simulink model "virtualWallSim"  (Simulink 8.1)
settings: Solver=ode45  StartTime=0.0  StopTime=5  MaxStep=0.01  RelTol=1e-3
libraries: simulink x1
settings Model: Creator=jasonyt  LastModifiedBy=jasonyt
settings DataIOCC: LimitDataPoints=off  SignalLoggingSaveFormat=Dataset
settings OptimizationCC: ExpressionDepthLimit=128
settings DebuggingCC: FcnCallInpInsideContextMsg=EnableAllAsError
settings GRTTargetCC: CombineOutputUpdateFcns=on  GRTInterface=off

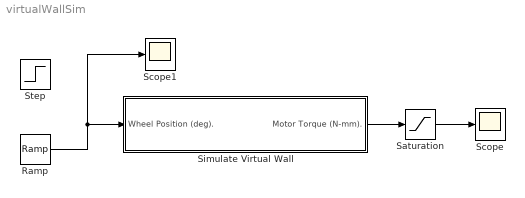
== system virtualWallSim ==
  Ramp : simulink/Sources/Ramp  slope=10  start=0  X0=-20
  Saturation : Saturate  UpperLimit=825  LowerLimit=-825
  Scope : Scope
  Scope1 : Scope
  Simulate Virtual Wall : Subsystem
  Step : Step  After=10  SampleTime=0
  wires:
  Simulate Virtual Wall/1(Motor Torque (N-mm).) -> Saturation/1
  Saturation/1 -> Scope/1
  Ramp/1 -> Scope1/1, Simulate Virtual Wall/1(Wheel Position (deg).)

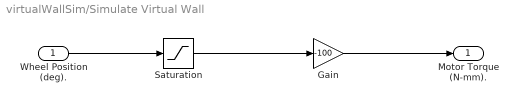
== system virtualWallSim/Simulate Virtual Wall ==
  Wheel Position (deg). : Inport
  Gain : Gain  Gain=-100
  Saturation : Saturate  UpperLimit=Inf  LowerLimit=0
  Motor Torque (N-mm). : Outport
  wires:
  Wheel Position (deg)./1 -> Saturation/1
  Saturation/1 -> Gain/1
  Gain/1 -> Motor Torque (N-mm)./1
